simulink model "sampleModel646original"  (R2021b)
settings: Solver=VariableStepAuto  StartTime=0.0  StopTime=10.0  RelTol=1e-3
undefined symbols (not defined in the file): DiscIntNeverNeededParam, Newton, Raphson, sigbuilder_block
libraries: simulink x194, slpidlib x27
(part 4 of 5)

== system sampleModel646original/emi_2124 ==
  In1 : Inport
  emi_2125 : Inport  Port=2
  emi_2127 : slpidlib/PID Controller  Controller=PID  Form=Parallel  TimeDomain=Discrete-time  UseExternalTs=off  SampleTime=-1  IntegratorMethod=Forward Euler  FilterMethod=Forward Euler  ControllerParametersSource=internal  P=1  I=1  D=0  UseFilter=on  N=100  TunerSelectOption=Transfer Function Based (PID Tuner App)  InitialConditionSource=internal  InitialConditionForIntegrator=0  InitialConditionForFilter=0  DifferentiatorICPrevScaledInput=0  ExternalReset=none  TrackingMode=off  Kt=1  LimitOutput=off  SatLimitsSource=internal  UpperSaturationLimit=inf  LowerSaturationLimit=-inf  LinearizeAsGain=off  AntiWindupMode=none  Kb=1  POutMin=[]  POutMax=[]  IOutMin=[]  IOutMax=[]  DOutMin=[]  DOutMax=[]  NOutMin=[]  NOutMax=[]  SumOutMin=[]  SumOutMax=[]  SaturationOutMin=[]  SaturationOutMax=[]  PParamMin=[]  PParamMax=[]  IParamMin=[]  IParamMax=[]  DParamMin=[]  DParamMax=[]  NParamMin=[]  NParamMax=[]  KbParamMin=[]  KbParamMax=[]  KtParamMin=[]  KtParamMax=[]  KbOutMin=[]  KbOutMax=[]  KtOutMin=[]  KtOutMax=[]  IntegratorOutMin=[]  IntegratorOutMax=[]  FilterOutMin=[]  FilterOutMax=[]  SumI1OutMin=[]  SumI1OutMax=[]  SumI2OutMin=[]  SumI2OutMax=[]  SumI3OutMin=[]  SumI3OutMax=[]  SumI4OutMin=[]  SumI4OutMax=[]  SumDOutMin=[]  SumDOutMax=[]  DifferentiatorOutMin=[]  DifferentiatorOutMax=[]  FilterDiffOutCoefMin=[]  FilterDiffOutCoefMax=[]  ReciprocalOutMin=[]  ReciprocalOutMax=[]  SumDenOutMin=[]  SumDenOutMax=[]  SumNumOutMin=[]  SumNumOutMax=[]  DivideOutMin=[]  DivideOutMax=[]  UdiffTsProdOutMin=[]  UdiffTsProdOutMax=[]  NTsProdOutMin=[]  NTsProdOutMax=[]  UintegralTsProdOutMin=[]  UintegralTsProdOutMax=[]  UngainTsProdOutMin=[]  UngainTsProdOutMax=[]  IntegratorContinuousStateAttributes=''  IntegratorStateMustResolveToSignalObject=off  IntegratorRTWStateStorageClass=Auto  FilterContinuousStateAttributes=''  FilterStateMustResolveToSignalObject=off  FilterRTWStateStorageClass=Auto  ParallelPVariant=InternalParameters  IdealPVariant=Disabled  IVariant=InternalParameters  DVariant=InternalParameters  IntegratorVariant=Discrete  SatVariant=Disabled  AWVariant=Passthrough  PCopyVariant=Disabled  TRVariant=Disabled  FdbkBlocksVariant=Forward  IdealPFdbkVariant=Disabled  SatFdbkVariant=Disabled  DerivativeFilterVariant=ForwardEulerFilter  NVariant=InternalParameters  NCopyVariant=Disabled  FilterICVariant=InternalICsFilter  IntegratorICVariant=InternalICs  ExternalResetVariant=Disabled  TRSumVariant=Passthrough  SumFdbkVariant=Disabled  SumVariant=Sum_PID  TsampFilterVariant=InternalTs  TsampNgainVariant=Passthrough  TsampIntegralVariant=Passthrough  ExternalSaturationOutDataTypeStr=Inherit: Same as second input
  emi_2128 : simulink/Discrete/Difference  ICPrevInput=0.0  OutMin=[]  OutMax=[]  OutDataType=fixdt(1, 16)  OutScaling=2^-10  DoSatur=off
  emi_2129 : Sin  TimeSource=Use external signal  SampleTime=0
  emi_2130 : DiscreteZeroPole  Poles=[0 0.5]  Gain=1  SampleTime=-1
  emi_2131 : DiscreteZeroPole  Poles=[0 0.5]  Gain=1  SampleTime=-1
  emi_2132 : Math  SaturateOnIntegerOverflow=on
  emi_2133 : Rounding
  emi_2134 : simulink/Discontinuities/Rate Limiter Dynamic
  emi_2135 : simulink/Sources/Band-Limited White Noise  Cov=[0.1]  Ts=0.1  seed=[23341]
  Out1 : Outport
  emi_2126 : Outport  Port=2
  wires:
  In1/1 -> Out1/1
  emi_2127/1 -> emi_2128/1
  emi_2128/1 -> emi_2129/1
  emi_2129/1 -> emi_2130/1
  emi_2130/1 -> emi_2131/1
  emi_2131/1 -> emi_2132/1
  emi_2132/1 -> emi_2133/1
  emi_2133/1 -> emi_2134/1
  emi_2135/1 -> emi_2127/1
  emi_2134/1 -> emi_2126/1

== system sampleModel646original/emi_2143 ==
  emi_2150 : Inport
  Action Port : ActionPort  ActionPortLabel=if(0 > u1)
  emi_2147 : Math  SaturateOnIntegerOverflow=on
  emi_2148 : MinMax
  emi_2149 : Trigonometry
  emi_2152 : UnaryMinus
  emi_2153 : Gain
  emi_2154 : Trigonometry
  emi_2155 : Ground
  emi_2151 : Outport
  wires:
  emi_2150/1 -> emi_2147/1
  emi_2147/1 -> emi_2148/1
  emi_2148/1 -> emi_2149/1
  emi_2152/1 -> emi_2153/1
  emi_2153/1 -> emi_2154/1
  emi_2155/1 -> emi_2152/1
  emi_2154/1 -> emi_2151/1

== system sampleModel646original/emi_2158 ==
  In1 : Inport
  emi_2159 : Inport  Port=2
  emi_2161 : DiscreteStateSpace  SampleTime=-1
  emi_2162 : Relay
  emi_2163 : simulink/Discrete/Transfer Fcn First Order  PoleZ=0.95  ICPrevOutput=0.0  DoSatur=off
  emi_2164 : VariablePulseGenerator  SampleTime=0.1
  emi_2165 : Sum  Inputs=+
  emi_2166 : DiscreteTransferFcn
  emi_2167 : Sum  Inputs=+
  emi_2168 : Product  Inputs=*
  emi_2169 : simulink/Discontinuities/Wrap To Zero  Threshold=255
      settings: SourceProductBaseCode=SL
  emi_2170 : Quantizer
  emi_2171 : Sum  Inputs=+
  emi_2172 : DiscreteTransferFcn
  emi_2173 : simulink/Sources/Repeating Sequence Interpolated  OutValues=[3 1 4 2 1].'  TimeValues=[0 0.1 0.5 0.6 1].'  LookUpMeth=Interpolation-Use End Values  tsamp=0.01  OutMin=[]  OutMax=[]  OutDataTypeStr=double  OutputDataTypeScalingMode=double  OutDataType=fixdt(0,8)  OutScaling=2^-10
  Out1 : Outport
  emi_2160 : Outport  Port=2
  wires:
  In1/1 -> Out1/1
  emi_2161/1 -> emi_2162/1
  emi_2162/1 -> emi_2163/1
  emi_2163/1 -> emi_2164/1
  emi_2164/1 -> emi_2165/1
  emi_2165/1 -> emi_2166/1
  emi_2166/1 -> emi_2167/1
  emi_2167/1 -> emi_2168/1
  emi_2168/1 -> emi_2169/1
  emi_2169/1 -> emi_2170/1
  emi_2170/1 -> emi_2171/1
  emi_2171/1 -> emi_2172/1
  emi_2173/1 -> emi_2161/1
  emi_2172/1 -> emi_2160/1

== system sampleModel646original/emi_2180 ==
  emi_2187 : Inport
  Action Port : ActionPort  ActionPortLabel=if(0 > u1)
  emi_2184 : Trigonometry
  emi_2185 : Math  SaturateOnIntegerOverflow=on
  emi_2186 : MinMax
  emi_2189 : Sum  Inputs=+
  emi_2190 : Ground
  emi_2188 : Outport
  wires:
  emi_2187/1 -> emi_2184/1
  emi_2184/1 -> emi_2185/1
  emi_2185/1 -> emi_2186/1
  emi_2190/1 -> emi_2189/1
  emi_2189/1 -> emi_2188/1

== system sampleModel646original/emi_2193 ==
  In1 : Inport
  emi_2194 : Inport  Port=2
  emi_2196 : DiscreteStateSpace  SampleTime=-1
  emi_2197 : Product  Inputs=*
  emi_2198 : simulink/Discontinuities/Wrap To Zero  Threshold=255
      settings: SourceProductBaseCode=SL
  emi_2199 : simulink/Discrete/Transfer Fcn First Order  PoleZ=0.95  ICPrevOutput=0.0  DoSatur=off
  emi_2200 : simulink/Discontinuities/PWM  DisableCoverage=on  Period=1  DisallowZeroDutyCycle=off  RunAtFixedTimeIntervals=off  SampleTime=0.1
  emi_2201 : Rounding
  emi_2202 : DeadZone  SaturateOnIntegerOverflow=on
  emi_2203 : Clock
  Out1 : Outport
  emi_2195 : Outport  Port=2
  wires:
  In1/1 -> Out1/1
  emi_2196/1 -> emi_2197/1
  emi_2197/1 -> emi_2198/1
  emi_2198/1 -> emi_2199/1
  emi_2199/1 -> emi_2200/1
  emi_2200/1 -> emi_2201/1
  emi_2201/1 -> emi_2202/1
  emi_2203/1 -> emi_2196/1
  emi_2202/1 -> emi_2195/1

== system sampleModel646original/emi_22 ==
  In1 : Inport
  emi_23 : Inport  Port=2
  emi_25 : DiscreteZeroPole  Poles=[0 0.5]  Gain=1  SampleTime=-1
  emi_26 : simulink/Discontinuities/Saturation Dynamic  OutMin=[]  OutMax=[]  OutDataTypeStr=Inherit: Same as second input  OutDataType=fixdt(1, 16)  OutScaling=2^-10  DoSatur=off
  emi_27 : Sqrt  Operator=rSqrt  SaturateOnIntegerOverflow=on
  emi_28 : Relay
  emi_29 : simulink/Discontinuities/Wrap To Zero  Threshold=255
      settings: SourceProductBaseCode=SL
  emi_30 : VariablePulseGenerator  SampleTime=0.1
  emi_31 : Math  SaturateOnIntegerOverflow=on
  emi_32 : DiscreteZeroPole  Poles=[0 0.5]  Gain=1  SampleTime=-1
  emi_33 : DiscreteIntegrator  SampleTime=-1  ICPrevOutput=DiscIntNeverNeededParam  ICPrevScaledInput=DiscIntNeverNeededParam
  emi_34 : DiscreteTransferFcn
  emi_35 : VariablePulseGenerator  SampleTime=0.1
  emi_36 : simulink/Discrete/Transfer Fcn First Order  PoleZ=0.95  ICPrevOutput=0.0  DoSatur=off
  emi_37 : slpidlib/PID Controller  Controller=PID  Form=Parallel  TimeDomain=Discrete-time  UseExternalTs=off  SampleTime=-1  IntegratorMethod=Forward Euler  FilterMethod=Forward Euler  ControllerParametersSource=internal  P=1  I=1  D=0  UseFilter=on  N=100  TunerSelectOption=Transfer Function Based (PID Tuner App)  InitialConditionSource=internal  InitialConditionForIntegrator=0  InitialConditionForFilter=0  DifferentiatorICPrevScaledInput=0  ExternalReset=none  TrackingMode=off  Kt=1  LimitOutput=off  SatLimitsSource=internal  UpperSaturationLimit=inf  LowerSaturationLimit=-inf  LinearizeAsGain=off  AntiWindupMode=none  Kb=1  POutMin=[]  POutMax=[]  IOutMin=[]  IOutMax=[]  DOutMin=[]  DOutMax=[]  NOutMin=[]  NOutMax=[]  SumOutMin=[]  SumOutMax=[]  SaturationOutMin=[]  SaturationOutMax=[]  PParamMin=[]  PParamMax=[]  IParamMin=[]  IParamMax=[]  DParamMin=[]  DParamMax=[]  NParamMin=[]  NParamMax=[]  KbParamMin=[]  KbParamMax=[]  KtParamMin=[]  KtParamMax=[]  KbOutMin=[]  KbOutMax=[]  KtOutMin=[]  KtOutMax=[]  IntegratorOutMin=[]  IntegratorOutMax=[]  FilterOutMin=[]  FilterOutMax=[]  SumI1OutMin=[]  SumI1OutMax=[]  SumI2OutMin=[]  SumI2OutMax=[]  SumI3OutMin=[]  SumI3OutMax=[]  SumI4OutMin=[]  SumI4OutMax=[]  SumDOutMin=[]  SumDOutMax=[]  DifferentiatorOutMin=[]  DifferentiatorOutMax=[]  FilterDiffOutCoefMin=[]  FilterDiffOutCoefMax=[]  ReciprocalOutMin=[]  ReciprocalOutMax=[]  SumDenOutMin=[]  SumDenOutMax=[]  SumNumOutMin=[]  SumNumOutMax=[]  DivideOutMin=[]  DivideOutMax=[]  UdiffTsProdOutMin=[]  UdiffTsProdOutMax=[]  NTsProdOutMin=[]  NTsProdOutMax=[]  UintegralTsProdOutMin=[]  UintegralTsProdOutMax=[]  UngainTsProdOutMin=[]  UngainTsProdOutMax=[]  IntegratorContinuousStateAttributes=''  IntegratorStateMustResolveToSignalObject=off  IntegratorRTWStateStorageClass=Auto  FilterContinuousStateAttributes=''  FilterStateMustResolveToSignalObject=off  FilterRTWStateStorageClass=Auto  ParallelPVariant=InternalParameters  IdealPVariant=Disabled  IVariant=InternalParameters  DVariant=InternalParameters  IntegratorVariant=Discrete  SatVariant=Disabled  AWVariant=Passthrough  PCopyVariant=Disabled  TRVariant=Disabled  FdbkBlocksVariant=Forward  IdealPFdbkVariant=Disabled  SatFdbkVariant=Disabled  DerivativeFilterVariant=ForwardEulerFilter  NVariant=InternalParameters  NCopyVariant=Disabled  FilterICVariant=InternalICsFilter  IntegratorICVariant=InternalICs  ExternalResetVariant=Disabled  TRSumVariant=Passthrough  SumFdbkVariant=Disabled  SumVariant=Sum_PID  TsampFilterVariant=InternalTs  TsampNgainVariant=Passthrough  TsampIntegralVariant=Passthrough  ExternalSaturationOutDataTypeStr=Inherit: Same as second input
  emi_38 : Abs
  emi_39 : Sum  Inputs=+
  emi_40 : UnaryMinus
  emi_41 : Sin  TimeSource=Use external signal  SampleTime=0
  emi_42 : Math  SaturateOnIntegerOverflow=on
  emi_43 : slpidlib/PID Controller  Controller=PID  Form=Parallel  TimeDomain=Discrete-time  UseExternalTs=off  SampleTime=-1  IntegratorMethod=Forward Euler  FilterMethod=Forward Euler  ControllerParametersSource=internal  P=1  I=1  D=0  UseFilter=on  N=100  TunerSelectOption=Transfer Function Based (PID Tuner App)  InitialConditionSource=internal  InitialConditionForIntegrator=0  InitialConditionForFilter=0  DifferentiatorICPrevScaledInput=0  ExternalReset=none  TrackingMode=off  Kt=1  LimitOutput=off  SatLimitsSource=internal  UpperSaturationLimit=inf  LowerSaturationLimit=-inf  LinearizeAsGain=off  AntiWindupMode=none  Kb=1  POutMin=[]  POutMax=[]  IOutMin=[]  IOutMax=[]  DOutMin=[]  DOutMax=[]  NOutMin=[]  NOutMax=[]  SumOutMin=[]  SumOutMax=[]  SaturationOutMin=[]  SaturationOutMax=[]  PParamMin=[]  PParamMax=[]  IParamMin=[]  IParamMax=[]  DParamMin=[]  DParamMax=[]  NParamMin=[]  NParamMax=[]  KbParamMin=[]  KbParamMax=[]  KtParamMin=[]  KtParamMax=[]  KbOutMin=[]  KbOutMax=[]  KtOutMin=[]  KtOutMax=[]  IntegratorOutMin=[]  IntegratorOutMax=[]  FilterOutMin=[]  FilterOutMax=[]  SumI1OutMin=[]  SumI1OutMax=[]  SumI2OutMin=[]  SumI2OutMax=[]  SumI3OutMin=[]  SumI3OutMax=[]  SumI4OutMin=[]  SumI4OutMax=[]  SumDOutMin=[]  SumDOutMax=[]  DifferentiatorOutMin=[]  DifferentiatorOutMax=[]  FilterDiffOutCoefMin=[]  FilterDiffOutCoefMax=[]  ReciprocalOutMin=[]  ReciprocalOutMax=[]  SumDenOutMin=[]  SumDenOutMax=[]  SumNumOutMin=[]  SumNumOutMax=[]  DivideOutMin=[]  DivideOutMax=[]  UdiffTsProdOutMin=[]  UdiffTsProdOutMax=[]  NTsProdOutMin=[]  NTsProdOutMax=[]  UintegralTsProdOutMin=[]  UintegralTsProdOutMax=[]  UngainTsProdOutMin=[]  UngainTsProdOutMax=[]  IntegratorContinuousStateAttributes=''  IntegratorStateMustResolveToSignalObject=off  IntegratorRTWStateStorageClass=Auto  FilterContinuousStateAttributes=''  FilterStateMustResolveToSignalObject=off  FilterRTWStateStorageClass=Auto  ParallelPVariant=InternalParameters  IdealPVariant=Disabled  IVariant=InternalParameters  DVariant=InternalParameters  IntegratorVariant=Discrete  SatVariant=Disabled  AWVariant=Passthrough  PCopyVariant=Disabled  TRVariant=Disabled  FdbkBlocksVariant=Forward  IdealPFdbkVariant=Disabled  SatFdbkVariant=Disabled  DerivativeFilterVariant=ForwardEulerFilter  NVariant=InternalParameters  NCopyVariant=Disabled  FilterICVariant=InternalICsFilter  IntegratorICVariant=InternalICs  ExternalResetVariant=Disabled  TRSumVariant=Passthrough  SumFdbkVariant=Disabled  SumVariant=Sum_PID  TsampFilterVariant=InternalTs  TsampNgainVariant=Passthrough  TsampIntegralVariant=Passthrough  ExternalSaturationOutDataTypeStr=Inherit: Same as second input
  emi_44 : Math  SaturateOnIntegerOverflow=on
  emi_45 : slpidlib/PID Controller  Controller=PID  Form=Parallel  TimeDomain=Discrete-time  UseExternalTs=off  SampleTime=-1  IntegratorMethod=Forward Euler  FilterMethod=Forward Euler  ControllerParametersSource=internal  P=1  I=1  D=0  UseFilter=on  N=100  TunerSelectOption=Transfer Function Based (PID Tuner App)  InitialConditionSource=internal  InitialConditionForIntegrator=0  InitialConditionForFilter=0  DifferentiatorICPrevScaledInput=0  ExternalReset=none  TrackingMode=off  Kt=1  LimitOutput=off  SatLimitsSource=internal  UpperSaturationLimit=inf  LowerSaturationLimit=-inf  LinearizeAsGain=off  AntiWindupMode=none  Kb=1  POutMin=[]  POutMax=[]  IOutMin=[]  IOutMax=[]  DOutMin=[]  DOutMax=[]  NOutMin=[]  NOutMax=[]  SumOutMin=[]  SumOutMax=[]  SaturationOutMin=[]  SaturationOutMax=[]  PParamMin=[]  PParamMax=[]  IParamMin=[]  IParamMax=[]  DParamMin=[]  DParamMax=[]  NParamMin=[]  NParamMax=[]  KbParamMin=[]  KbParamMax=[]  KtParamMin=[]  KtParamMax=[]  KbOutMin=[]  KbOutMax=[]  KtOutMin=[]  KtOutMax=[]  IntegratorOutMin=[]  IntegratorOutMax=[]  FilterOutMin=[]  FilterOutMax=[]  SumI1OutMin=[]  SumI1OutMax=[]  SumI2OutMin=[]  SumI2OutMax=[]  SumI3OutMin=[]  SumI3OutMax=[]  SumI4OutMin=[]  SumI4OutMax=[]  SumDOutMin=[]  SumDOutMax=[]  DifferentiatorOutMin=[]  DifferentiatorOutMax=[]  FilterDiffOutCoefMin=[]  FilterDiffOutCoefMax=[]  ReciprocalOutMin=[]  ReciprocalOutMax=[]  SumDenOutMin=[]  SumDenOutMax=[]  SumNumOutMin=[]  SumNumOutMax=[]  DivideOutMin=[]  DivideOutMax=[]  UdiffTsProdOutMin=[]  UdiffTsProdOutMax=[]  NTsProdOutMin=[]  NTsProdOutMax=[]  UintegralTsProdOutMin=[]  UintegralTsProdOutMax=[]  UngainTsProdOutMin=[]  UngainTsProdOutMax=[]  IntegratorContinuousStateAttributes=''  IntegratorStateMustResolveToSignalObject=off  IntegratorRTWStateStorageClass=Auto  FilterContinuousStateAttributes=''  FilterStateMustResolveToSignalObject=off  FilterRTWStateStorageClass=Auto  ParallelPVariant=InternalParameters  IdealPVariant=Disabled  IVariant=InternalParameters  DVariant=InternalParameters  IntegratorVariant=Discrete  SatVariant=Disabled  AWVariant=Passthrough  PCopyVariant=Disabled  TRVariant=Disabled  FdbkBlocksVariant=Forward  IdealPFdbkVariant=Disabled  SatFdbkVariant=Disabled  DerivativeFilterVariant=ForwardEulerFilter  NVariant=InternalParameters  NCopyVariant=Disabled  FilterICVariant=InternalICsFilter  IntegratorICVariant=InternalICs  ExternalResetVariant=Disabled  TRSumVariant=Passthrough  SumFdbkVariant=Disabled  SumVariant=Sum_PID  TsampFilterVariant=InternalTs  TsampNgainVariant=Passthrough  TsampIntegralVariant=Passthrough  ExternalSaturationOutDataTypeStr=Inherit: Same as second input
  emi_46 : DiscreteFir
  emi_47 : VariablePulseGenerator  SampleTime=0.1
  emi_48 : Sum  Inputs=+
  emi_49 : simulink/Discrete/Transfer Fcn First Order  PoleZ=0.95  ICPrevOutput=0.0  DoSatur=off
  emi_50 : Quantizer
  emi_51 : DiscreteTransferFcn
  emi_52 : Sin  TimeSource=Use external signal  SampleTime=0
  emi_53 : simulink/Discontinuities/PWM  DisableCoverage=on  Period=1  DisallowZeroDutyCycle=off  RunAtFixedTimeIntervals=off  SampleTime=0.1
  emi_54 : simulink/Sources/Repeating Sequence  rep_seq_t=[0 2]  rep_seq_y=[0 2]
  Out1 : Outport
  emi_24 : Outport  Port=2
  wires:
  In1/1 -> Out1/1
  emi_25/1 -> emi_26/1
  emi_26/1 -> emi_27/1
  emi_27/1 -> emi_28/1
  emi_28/1 -> emi_29/1
  emi_29/1 -> emi_30/1
  emi_30/1 -> emi_31/1
  emi_31/1 -> emi_32/1
  emi_32/1 -> emi_33/1
  emi_33/1 -> emi_34/1
  emi_34/1 -> emi_35/1
  emi_35/1 -> emi_36/1
  emi_36/1 -> emi_37/1
  emi_37/1 -> emi_38/1
  emi_38/1 -> emi_39/1
  emi_39/1 -> emi_40/1
  emi_40/1 -> emi_41/1
  emi_41/1 -> emi_42/1
  emi_42/1 -> emi_43/1
  emi_43/1 -> emi_44/1
  emi_44/1 -> emi_45/1
  emi_45/1 -> emi_46/1
  emi_46/1 -> emi_47/1
  emi_47/1 -> emi_48/1
  emi_48/1 -> emi_49/1
  emi_49/1 -> emi_50/1
  emi_50/1 -> emi_51/1
  emi_51/1 -> emi_52/1
  emi_52/1 -> emi_53/1
  emi_54/1 -> emi_25/1
  emi_53/1 -> emi_24/1

== system sampleModel646original/emi_2210 ==
  emi_2217 : Inport
  Action Port : ActionPort  ActionPortLabel=if(0 > u1)
  emi_{2214,2216,2228,2238} (4 alike) : Gain
  emi_2215 : Abs
  emi_2219 : Trigonometry
  emi_2220 : Trigonometry
  emi_{2221,2223,2227,2233,2235,2239} (6 alike) : Sin  TimeSource=Use external signal  SampleTime=0
  emi_2222 : Product  Inputs=*
  emi_2224 : Math  SaturateOnIntegerOverflow=on
  emi_2225 : Math  SaturateOnIntegerOverflow=on
  emi_2226 : Sum  Inputs=+
  emi_2229 : MinMax
  emi_2230 : Product  Inputs=*
  emi_2231 : Sqrt  Operator=rSqrt  SaturateOnIntegerOverflow=on
  emi_2232 : Math  SaturateOnIntegerOverflow=on
  emi_2234 : Abs
  emi_2236 : Sum  Inputs=+
  emi_2237 : Sqrt  Operator=rSqrt  SaturateOnIntegerOverflow=on
  emi_2240 : Sum  Inputs=+
  emi_2241 : Ground
  emi_2218 : Outport
  wires:
  emi_2217/1 -> emi_2214/1
  emi_2214/1 -> emi_2215/1
  emi_2215/1 -> emi_2216/1
  emi_2219/1 -> emi_2220/1
  emi_2220/1 -> emi_2221/1
  emi_2221/1 -> emi_2222/1
  emi_2222/1 -> emi_2223/1
  emi_2223/1 -> emi_2224/1
  emi_2224/1 -> emi_2225/1
  emi_2225/1 -> emi_2226/1
  emi_2226/1 -> emi_2227/1
  emi_2227/1 -> emi_2228/1
  emi_2228/1 -> emi_2229/1
  emi_2229/1 -> emi_2230/1
  emi_2230/1 -> emi_2231/1
  emi_2231/1 -> emi_2232/1
  emi_2232/1 -> emi_2233/1
  emi_2233/1 -> emi_2234/1
  emi_2234/1 -> emi_2235/1
  emi_2235/1 -> emi_2236/1
  emi_2236/1 -> emi_2237/1
  emi_2237/1 -> emi_2238/1
  emi_2238/1 -> emi_2239/1
  emi_2239/1 -> emi_2240/1
  emi_2241/1 -> emi_2219/1
  emi_2240/1 -> emi_2218/1

== system sampleModel646original/emi_2244 ==
  In1 : Inport
  emi_2245 : Inport  Port=2
  emi_2247 : UnaryMinus
  emi_2248 : simulink/Discontinuities/Saturation Dynamic  OutMin=[]  OutMax=[]  OutDataTypeStr=Inherit: Same as second input  OutDataType=fixdt(1, 16)  OutScaling=2^-10  DoSatur=off
  emi_2249 : Product  Inputs=*
  emi_2250 : Abs
  emi_2251 : simulink/Discontinuities/Saturation Dynamic  OutMin=[]  OutMax=[]  OutDataTypeStr=Inherit: Same as second input  OutDataType=fixdt(1, 16)  OutScaling=2^-10  DoSatur=off
  emi_2252 : slpidlib/PID Controller  Controller=PID  Form=Parallel  TimeDomain=Discrete-time  UseExternalTs=off  SampleTime=-1  IntegratorMethod=Forward Euler  FilterMethod=Forward Euler  ControllerParametersSource=internal  P=1  I=1  D=0  UseFilter=on  N=100  TunerSelectOption=Transfer Function Based (PID Tuner App)  InitialConditionSource=internal  InitialConditionForIntegrator=0  InitialConditionForFilter=0  DifferentiatorICPrevScaledInput=0  ExternalReset=none  TrackingMode=off  Kt=1  LimitOutput=off  SatLimitsSource=internal  UpperSaturationLimit=inf  LowerSaturationLimit=-inf  LinearizeAsGain=off  AntiWindupMode=none  Kb=1  POutMin=[]  POutMax=[]  IOutMin=[]  IOutMax=[]  DOutMin=[]  DOutMax=[]  NOutMin=[]  NOutMax=[]  SumOutMin=[]  SumOutMax=[]  SaturationOutMin=[]  SaturationOutMax=[]  PParamMin=[]  PParamMax=[]  IParamMin=[]  IParamMax=[]  DParamMin=[]  DParamMax=[]  NParamMin=[]  NParamMax=[]  KbParamMin=[]  KbParamMax=[]  KtParamMin=[]  KtParamMax=[]  KbOutMin=[]  KbOutMax=[]  KtOutMin=[]  KtOutMax=[]  IntegratorOutMin=[]  IntegratorOutMax=[]  FilterOutMin=[]  FilterOutMax=[]  SumI1OutMin=[]  SumI1OutMax=[]  SumI2OutMin=[]  SumI2OutMax=[]  SumI3OutMin=[]  SumI3OutMax=[]  SumI4OutMin=[]  SumI4OutMax=[]  SumDOutMin=[]  SumDOutMax=[]  DifferentiatorOutMin=[]  DifferentiatorOutMax=[]  FilterDiffOutCoefMin=[]  FilterDiffOutCoefMax=[]  ReciprocalOutMin=[]  ReciprocalOutMax=[]  SumDenOutMin=[]  SumDenOutMax=[]  SumNumOutMin=[]  SumNumOutMax=[]  DivideOutMin=[]  DivideOutMax=[]  UdiffTsProdOutMin=[]  UdiffTsProdOutMax=[]  NTsProdOutMin=[]  NTsProdOutMax=[]  UintegralTsProdOutMin=[]  UintegralTsProdOutMax=[]  UngainTsProdOutMin=[]  UngainTsProdOutMax=[]  IntegratorContinuousStateAttributes=''  IntegratorStateMustResolveToSignalObject=off  IntegratorRTWStateStorageClass=Auto  FilterContinuousStateAttributes=''  FilterStateMustResolveToSignalObject=off  FilterRTWStateStorageClass=Auto  ParallelPVariant=InternalParameters  IdealPVariant=Disabled  IVariant=InternalParameters  DVariant=InternalParameters  IntegratorVariant=Discrete  SatVariant=Disabled  AWVariant=Passthrough  PCopyVariant=Disabled  TRVariant=Disabled  FdbkBlocksVariant=Forward  IdealPFdbkVariant=Disabled  SatFdbkVariant=Disabled  DerivativeFilterVariant=ForwardEulerFilter  NVariant=InternalParameters  NCopyVariant=Disabled  FilterICVariant=InternalICsFilter  IntegratorICVariant=InternalICs  ExternalResetVariant=Disabled  TRSumVariant=Passthrough  SumFdbkVariant=Disabled  SumVariant=Sum_PID  TsampFilterVariant=InternalTs  TsampNgainVariant=Passthrough  TsampIntegralVariant=Passthrough  ExternalSaturationOutDataTypeStr=Inherit: Same as second input
  emi_2253 : Trigonometry
  emi_2254 : DiscreteFir
  emi_2255 : Rounding
  emi_2256 : Rounding
  emi_2257 : Rounding
  emi_2258 : DiscreteTransferFcn
  emi_2259 : Relay
  emi_2260 : Sin  TimeSource=Use external signal  SampleTime=0
  emi_2261 : simulink/Sources/Repeating Sequence Stair  OutValues=[3 1 4 2 1].'  tsamp=-1  OutMin=[]  OutMax=[]  OutDataTypeStr=double  OutputDataTypeScalingMode=double  OutDataType=fixdt(0,8)  ConRadixGroup=Best Precision: Vector-wise  OutScaling=2^-12
  Out1 : Outport
  emi_2246 : Outport  Port=2
  wires:
  In1/1 -> Out1/1
  emi_2247/1 -> emi_2248/1
  emi_2248/1 -> emi_2249/1
  emi_2249/1 -> emi_2250/1
  emi_2250/1 -> emi_2251/1
  emi_2251/1 -> emi_2252/1
  emi_2252/1 -> emi_2253/1
  emi_2253/1 -> emi_2254/1
  emi_2254/1 -> emi_2255/1
  emi_2255/1 -> emi_2256/1
  emi_2256/1 -> emi_2257/1
  emi_2257/1 -> emi_2258/1
  emi_2258/1 -> emi_2259/1
  emi_2259/1 -> emi_2260/1
  emi_2261/1 -> emi_2247/1
  emi_2260/1 -> emi_2246/1

== system sampleModel646original/emi_231 ==
  In1 : Inport
  emi_232 : Inport  Port=2
  emi_234 : Relay
  emi_235 : simulink/Discontinuities/Rate Limiter Dynamic
  emi_236 : DiscreteZeroPole  Poles=[0 0.5]  Gain=1  SampleTime=-1
  emi_237 : slpidlib/PID Controller  Controller=PID  Form=Parallel  TimeDomain=Discrete-time  UseExternalTs=off  SampleTime=-1  IntegratorMethod=Forward Euler  FilterMethod=Forward Euler  ControllerParametersSource=internal  P=1  I=1  D=0  UseFilter=on  N=100  TunerSelectOption=Transfer Function Based (PID Tuner App)  InitialConditionSource=internal  InitialConditionForIntegrator=0  InitialConditionForFilter=0  DifferentiatorICPrevScaledInput=0  ExternalReset=none  TrackingMode=off  Kt=1  LimitOutput=off  SatLimitsSource=internal  UpperSaturationLimit=inf  LowerSaturationLimit=-inf  LinearizeAsGain=off  AntiWindupMode=none  Kb=1  POutMin=[]  POutMax=[]  IOutMin=[]  IOutMax=[]  DOutMin=[]  DOutMax=[]  NOutMin=[]  NOutMax=[]  SumOutMin=[]  SumOutMax=[]  SaturationOutMin=[]  SaturationOutMax=[]  PParamMin=[]  PParamMax=[]  IParamMin=[]  IParamMax=[]  DParamMin=[]  DParamMax=[]  NParamMin=[]  NParamMax=[]  KbParamMin=[]  KbParamMax=[]  KtParamMin=[]  KtParamMax=[]  KbOutMin=[]  KbOutMax=[]  KtOutMin=[]  KtOutMax=[]  IntegratorOutMin=[]  IntegratorOutMax=[]  FilterOutMin=[]  FilterOutMax=[]  SumI1OutMin=[]  SumI1OutMax=[]  SumI2OutMin=[]  SumI2OutMax=[]  SumI3OutMin=[]  SumI3OutMax=[]  SumI4OutMin=[]  SumI4OutMax=[]  SumDOutMin=[]  SumDOutMax=[]  DifferentiatorOutMin=[]  DifferentiatorOutMax=[]  FilterDiffOutCoefMin=[]  FilterDiffOutCoefMax=[]  ReciprocalOutMin=[]  ReciprocalOutMax=[]  SumDenOutMin=[]  SumDenOutMax=[]  SumNumOutMin=[]  SumNumOutMax=[]  DivideOutMin=[]  DivideOutMax=[]  UdiffTsProdOutMin=[]  UdiffTsProdOutMax=[]  NTsProdOutMin=[]  NTsProdOutMax=[]  UintegralTsProdOutMin=[]  UintegralTsProdOutMax=[]  UngainTsProdOutMin=[]  UngainTsProdOutMax=[]  IntegratorContinuousStateAttributes=''  IntegratorStateMustResolveToSignalObject=off  IntegratorRTWStateStorageClass=Auto  FilterContinuousStateAttributes=''  FilterStateMustResolveToSignalObject=off  FilterRTWStateStorageClass=Auto  ParallelPVariant=InternalParameters  IdealPVariant=Disabled  IVariant=InternalParameters  DVariant=InternalParameters  IntegratorVariant=Discrete  SatVariant=Disabled  AWVariant=Passthrough  PCopyVariant=Disabled  TRVariant=Disabled  FdbkBlocksVariant=Forward  IdealPFdbkVariant=Disabled  SatFdbkVariant=Disabled  DerivativeFilterVariant=ForwardEulerFilter  NVariant=InternalParameters  NCopyVariant=Disabled  FilterICVariant=InternalICsFilter  IntegratorICVariant=InternalICs  ExternalResetVariant=Disabled  TRSumVariant=Passthrough  SumFdbkVariant=Disabled  SumVariant=Sum_PID  TsampFilterVariant=InternalTs  TsampNgainVariant=Passthrough  TsampIntegralVariant=Passthrough  ExternalSaturationOutDataTypeStr=Inherit: Same as second input
  emi_238 : VariablePulseGenerator  SampleTime=0.1
  emi_239 : DiscreteStateSpace  SampleTime=-1
  emi_240 : Product  Inputs=*
  emi_241 : Sin  TimeSource=Use external signal  SampleTime=0
  emi_242 : Rounding
  emi_243 : MinMax
  emi_244 : simulink/Discrete/Transfer Fcn First Order  PoleZ=0.95  ICPrevOutput=0.0  DoSatur=off
  emi_245 : simulink/Discontinuities/Wrap To Zero  Threshold=255
      settings: SourceProductBaseCode=SL
  emi_246 : Math  SaturateOnIntegerOverflow=on
  emi_247 : simulink/Sources/Repeating Sequence Stair  OutValues=[3 1 4 2 1].'  tsamp=-1  OutMin=[]  OutMax=[]  OutDataTypeStr=double  OutputDataTypeScalingMode=double  OutDataType=fixdt(0,8)  ConRadixGroup=Best Precision: Vector-wise  OutScaling=2^-12
  Out1 : Outport
  emi_233 : Outport  Port=2
  wires:
  In1/1 -> Out1/1
  emi_234/1 -> emi_235/1
  emi_235/1 -> emi_236/1
  emi_236/1 -> emi_237/1
  emi_237/1 -> emi_238/1
  emi_238/1 -> emi_239/1
  emi_239/1 -> emi_240/1
  emi_240/1 -> emi_241/1
  emi_241/1 -> emi_242/1
  emi_242/1 -> emi_243/1
  emi_243/1 -> emi_244/1
  emi_244/1 -> emi_245/1
  emi_245/1 -> emi_246/1
  emi_247/1 -> emi_234/1
  emi_246/1 -> emi_233/1

== system sampleModel646original/emi_254 ==
  emi_261 : Inport
  Action Port : ActionPort  ActionPortLabel=if(-1.617560e+02 > u1)
  emi_258 : Trigonometry  SampleTime=1
  emi_259 : Math  SampleTime=1  SaturateOnIntegerOverflow=on
  emi_260 : Abs  SampleTime=1
  emi_263 : Abs
  emi_{264,270..271,275,287..288} (6 alike) : Product  Inputs=*
  emi_{265,284,286,289} (4 alike) : Sin  TimeSource=Use external signal  SampleTime=0
  emi_266 : UnaryMinus
  emi_267 : Abs
  emi_268 : UnaryMinus
  emi_{269,279..280,283,285,290} (6 alike) : Sqrt  Operator=rSqrt  SaturateOnIntegerOverflow=on
  emi_272 : MinMax
  emi_273 : Sum  Inputs=+
  emi_274 : UnaryMinus
  emi_276 : Sum  Inputs=+
  emi_277 : Math  SaturateOnIntegerOverflow=on
  emi_278 : Math  SaturateOnIntegerOverflow=on
  emi_281 : Abs
  emi_282 : Rounding
  emi_291 : MinMax
  emi_292 : MinMax
  emi_293 : Gain
  emi_294 : Gain
  emi_295 : Ground
  emi_262 : Outport
  wires:
  emi_261/1 -> emi_258/1
  emi_258/1 -> emi_259/1
  emi_259/1 -> emi_260/1
  emi_263/1 -> emi_264/1
  emi_264/1 -> emi_265/1
  emi_265/1 -> emi_266/1
  emi_266/1 -> emi_267/1
  emi_267/1 -> emi_268/1
  emi_268/1 -> emi_269/1
  emi_269/1 -> emi_270/1
  emi_270/1 -> emi_271/1
  emi_271/1 -> emi_272/1
  emi_272/1 -> emi_273/1
  emi_273/1 -> emi_274/1
  emi_274/1 -> emi_275/1
  emi_275/1 -> emi_276/1
  emi_276/1 -> emi_277/1
  emi_277/1 -> emi_278/1
  emi_278/1 -> emi_279/1
  emi_279/1 -> emi_280/1
  emi_280/1 -> emi_281/1
  emi_281/1 -> emi_282/1
  emi_282/1 -> emi_283/1
  emi_283/1 -> emi_284/1
  emi_284/1 -> emi_285/1
  emi_285/1 -> emi_286/1
  emi_286/1 -> emi_287/1
  emi_287/1 -> emi_288/1
  emi_288/1 -> emi_289/1
  emi_289/1 -> emi_290/1
  emi_290/1 -> emi_291/1
  emi_291/1 -> emi_292/1
  emi_292/1 -> emi_293/1
  emi_293/1 -> emi_294/1
  emi_295/1 -> emi_263/1
  emi_294/1 -> emi_262/1

== system sampleModel646original/emi_298 ==
  In1 : Inport
  emi_299 : Inport  Port=2
  emi_301 : DiscreteStateSpace  SampleTime=-1
  emi_302 : Math  SaturateOnIntegerOverflow=on
  emi_303 : Trigonometry
  emi_304 : simulink/Discontinuities/Rate Limiter Dynamic
  emi_305 : Quantizer
  emi_306 : VariablePulseGenerator  SampleTime=0.1
  emi_307 : DiscreteFir
  emi_308 : DiscreteTransferFcn
  emi_309 : Rounding
  emi_310 : DiscreteZeroPole  Poles=[0 0.5]  Gain=1  SampleTime=-1
  emi_311 : DiscreteFilter
  emi_312 : DeadZone  SaturateOnIntegerOverflow=on
  emi_313 : simulink/Discrete/Difference  ICPrevInput=0.0  OutMin=[]  OutMax=[]  OutDataType=fixdt(1, 16)  OutScaling=2^-10  DoSatur=off
  emi_314 : Sin  TimeSource=Use external signal  SampleTime=0
  emi_315 : DeadZone  SaturateOnIntegerOverflow=on
  emi_316 : Rounding
  emi_317 : Product  Inputs=*
  emi_318 : slpidlib/PID Controller  Controller=PID  Form=Parallel  TimeDomain=Discrete-time  UseExternalTs=off  SampleTime=-1  IntegratorMethod=Forward Euler  FilterMethod=Forward Euler  ControllerParametersSource=internal  P=1  I=1  D=0  UseFilter=on  N=100  TunerSelectOption=Transfer Function Based (PID Tuner App)  InitialConditionSource=internal  InitialConditionForIntegrator=0  InitialConditionForFilter=0  DifferentiatorICPrevScaledInput=0  ExternalReset=none  TrackingMode=off  Kt=1  LimitOutput=off  SatLimitsSource=internal  UpperSaturationLimit=inf  LowerSaturationLimit=-inf  LinearizeAsGain=off  AntiWindupMode=none  Kb=1  POutMin=[]  POutMax=[]  IOutMin=[]  IOutMax=[]  DOutMin=[]  DOutMax=[]  NOutMin=[]  NOutMax=[]  SumOutMin=[]  SumOutMax=[]  SaturationOutMin=[]  SaturationOutMax=[]  PParamMin=[]  PParamMax=[]  IParamMin=[]  IParamMax=[]  DParamMin=[]  DParamMax=[]  NParamMin=[]  NParamMax=[]  KbParamMin=[]  KbParamMax=[]  KtParamMin=[]  KtParamMax=[]  KbOutMin=[]  KbOutMax=[]  KtOutMin=[]  KtOutMax=[]  IntegratorOutMin=[]  IntegratorOutMax=[]  FilterOutMin=[]  FilterOutMax=[]  SumI1OutMin=[]  SumI1OutMax=[]  SumI2OutMin=[]  SumI2OutMax=[]  SumI3OutMin=[]  SumI3OutMax=[]  SumI4OutMin=[]  SumI4OutMax=[]  SumDOutMin=[]  SumDOutMax=[]  DifferentiatorOutMin=[]  DifferentiatorOutMax=[]  FilterDiffOutCoefMin=[]  FilterDiffOutCoefMax=[]  ReciprocalOutMin=[]  ReciprocalOutMax=[]  SumDenOutMin=[]  SumDenOutMax=[]  SumNumOutMin=[]  SumNumOutMax=[]  DivideOutMin=[]  DivideOutMax=[]  UdiffTsProdOutMin=[]  UdiffTsProdOutMax=[]  NTsProdOutMin=[]  NTsProdOutMax=[]  UintegralTsProdOutMin=[]  UintegralTsProdOutMax=[]  UngainTsProdOutMin=[]  UngainTsProdOutMax=[]  IntegratorContinuousStateAttributes=''  IntegratorStateMustResolveToSignalObject=off  IntegratorRTWStateStorageClass=Auto  FilterContinuousStateAttributes=''  FilterStateMustResolveToSignalObject=off  FilterRTWStateStorageClass=Auto  ParallelPVariant=InternalParameters  IdealPVariant=Disabled  IVariant=InternalParameters  DVariant=InternalParameters  IntegratorVariant=Discrete  SatVariant=Disabled  AWVariant=Passthrough  PCopyVariant=Disabled  TRVariant=Disabled  FdbkBlocksVariant=Forward  IdealPFdbkVariant=Disabled  SatFdbkVariant=Disabled  DerivativeFilterVariant=ForwardEulerFilter  NVariant=InternalParameters  NCopyVariant=Disabled  FilterICVariant=InternalICsFilter  IntegratorICVariant=InternalICs  ExternalResetVariant=Disabled  TRSumVariant=Passthrough  SumFdbkVariant=Disabled  SumVariant=Sum_PID  TsampFilterVariant=InternalTs  TsampNgainVariant=Passthrough  TsampIntegralVariant=Passthrough  ExternalSaturationOutDataTypeStr=Inherit: Same as second input
  emi_319 : Sum  Inputs=+
  emi_320 : Rounding
  emi_321 : slpidlib/PID Controller  Controller=PID  Form=Parallel  TimeDomain=Discrete-time  UseExternalTs=off  SampleTime=-1  IntegratorMethod=Forward Euler  FilterMethod=Forward Euler  ControllerParametersSource=internal  P=1  I=1  D=0  UseFilter=on  N=100  TunerSelectOption=Transfer Function Based (PID Tuner App)  InitialConditionSource=internal  InitialConditionForIntegrator=0  InitialConditionForFilter=0  DifferentiatorICPrevScaledInput=0  ExternalReset=none  TrackingMode=off  Kt=1  LimitOutput=off  SatLimitsSource=internal  UpperSaturationLimit=inf  LowerSaturationLimit=-inf  LinearizeAsGain=off  AntiWindupMode=none  Kb=1  POutMin=[]  POutMax=[]  IOutMin=[]  IOutMax=[]  DOutMin=[]  DOutMax=[]  NOutMin=[]  NOutMax=[]  SumOutMin=[]  SumOutMax=[]  SaturationOutMin=[]  SaturationOutMax=[]  PParamMin=[]  PParamMax=[]  IParamMin=[]  IParamMax=[]  DParamMin=[]  DParamMax=[]  NParamMin=[]  NParamMax=[]  KbParamMin=[]  KbParamMax=[]  KtParamMin=[]  KtParamMax=[]  KbOutMin=[]  KbOutMax=[]  KtOutMin=[]  KtOutMax=[]  IntegratorOutMin=[]  IntegratorOutMax=[]  FilterOutMin=[]  FilterOutMax=[]  SumI1OutMin=[]  SumI1OutMax=[]  SumI2OutMin=[]  SumI2OutMax=[]  SumI3OutMin=[]  SumI3OutMax=[]  SumI4OutMin=[]  SumI4OutMax=[]  SumDOutMin=[]  SumDOutMax=[]  DifferentiatorOutMin=[]  DifferentiatorOutMax=[]  FilterDiffOutCoefMin=[]  FilterDiffOutCoefMax=[]  ReciprocalOutMin=[]  ReciprocalOutMax=[]  SumDenOutMin=[]  SumDenOutMax=[]  SumNumOutMin=[]  SumNumOutMax=[]  DivideOutMin=[]  DivideOutMax=[]  UdiffTsProdOutMin=[]  UdiffTsProdOutMax=[]  NTsProdOutMin=[]  NTsProdOutMax=[]  UintegralTsProdOutMin=[]  UintegralTsProdOutMax=[]  UngainTsProdOutMin=[]  UngainTsProdOutMax=[]  IntegratorContinuousStateAttributes=''  IntegratorStateMustResolveToSignalObject=off  IntegratorRTWStateStorageClass=Auto  FilterContinuousStateAttributes=''  FilterStateMustResolveToSignalObject=off  FilterRTWStateStorageClass=Auto  ParallelPVariant=InternalParameters  IdealPVariant=Disabled  IVariant=InternalParameters  DVariant=InternalParameters  IntegratorVariant=Discrete  SatVariant=Disabled  AWVariant=Passthrough  PCopyVariant=Disabled  TRVariant=Disabled  FdbkBlocksVariant=Forward  IdealPFdbkVariant=Disabled  SatFdbkVariant=Disabled  DerivativeFilterVariant=ForwardEulerFilter  NVariant=InternalParameters  NCopyVariant=Disabled  FilterICVariant=InternalICsFilter  IntegratorICVariant=InternalICs  ExternalResetVariant=Disabled  TRSumVariant=Passthrough  SumFdbkVariant=Disabled  SumVariant=Sum_PID  TsampFilterVariant=InternalTs  TsampNgainVariant=Passthrough  TsampIntegralVariant=Passthrough  ExternalSaturationOutDataTypeStr=Inherit: Same as second input
  emi_322 : Gain
  emi_323 : simulink/Discrete/Discrete Derivative  gainval=1.0  ICPrevScaledInput=0.0  OutMin=[]  OutMax=[]  OutDataType=fixdt(1, 16)  OutScaling=2^-10  DoSatur=off
  emi_324 : simulink/Discrete/Transfer Fcn First Order  PoleZ=0.95  ICPrevOutput=0.0  DoSatur=off
  emi_325 : Ground
  Out1 : Outport
  emi_300 : Outport  Port=2
  wires:
  In1/1 -> Out1/1
  emi_301/1 -> emi_302/1
  emi_302/1 -> emi_303/1
  emi_303/1 -> emi_304/1
  emi_304/1 -> emi_305/1
  emi_305/1 -> emi_306/1
  emi_306/1 -> emi_307/1
  emi_307/1 -> emi_308/1
  emi_308/1 -> emi_309/1
  emi_309/1 -> emi_310/1
  emi_310/1 -> emi_311/1
  emi_311/1 -> emi_312/1
  emi_312/1 -> emi_313/1
  emi_313/1 -> emi_314/1
  emi_314/1 -> emi_315/1
  emi_315/1 -> emi_316/1
  emi_316/1 -> emi_317/1
  emi_317/1 -> emi_318/1
  emi_318/1 -> emi_319/1
  emi_319/1 -> emi_320/1
  emi_320/1 -> emi_321/1
  emi_321/1 -> emi_322/1
  emi_322/1 -> emi_323/1
  emi_323/1 -> emi_324/1
  emi_325/1 -> emi_301/1
  emi_324/1 -> emi_300/1

== system sampleModel646original/emi_3 ==
  emi_10 : Inport
  Action Port : ActionPort  ActionPortLabel=if(-1.382844e+09 > u1)
  emi_12 : Sin  TimeSource=Use external signal  SampleTime=0
  emi_13 : Sum  Inputs=+
  emi_14 : Sqrt  Operator=rSqrt  SaturateOnIntegerOverflow=on
  emi_15 : Sin  TimeSource=Use external signal  SampleTime=0
  emi_16 : Trigonometry
  emi_17 : Sin  TimeSource=Use external signal  SampleTime=0
  emi_18 : Gain
  emi_19 : Ground
  emi_7 : Math  SampleTime=1  SaturateOnIntegerOverflow=on
  emi_8 : Abs  SampleTime=1
  emi_9 : Gain  SampleTime=1
  emi_11 : Outport
  wires:
  emi_10/1 -> emi_7/1
  emi_7/1 -> emi_8/1
  emi_8/1 -> emi_9/1
  emi_12/1 -> emi_13/1
  emi_13/1 -> emi_14/1
  emi_14/1 -> emi_15/1
  emi_15/1 -> emi_16/1
  emi_16/1 -> emi_17/1
  emi_17/1 -> emi_18/1
  emi_19/1 -> emi_12/1
  emi_18/1 -> emi_11/1

== system sampleModel646original/emi_332 ==
  emi_339 : Inport
  Action Port : ActionPort  ActionPortLabel=if(0 > u1)
  emi_336 : Gain  SampleTime=0
  emi_337 : MinMax  SampleTime=0
  emi_338 : Gain  SampleTime=0
  emi_341 : Sum  Inputs=+
  emi_{342,346,350,359} (4 alike) : Math  SaturateOnIntegerOverflow=on
  emi_343 : Trigonometry
  emi_344 : Trigonometry
  emi_345 : Trigonometry
  emi_347 : Product  Inputs=*
  emi_348 : Sin  TimeSource=Use external signal  SampleTime=0
  emi_349 : MinMax
  emi_351 : Gain
  emi_352 : Sqrt  Operator=rSqrt  SaturateOnIntegerOverflow=on
  emi_{353,357..358,363} (4 alike) : UnaryMinus
  emi_354 : MinMax
  emi_355 : Sqrt  Operator=rSqrt  SaturateOnIntegerOverflow=on
  emi_356 : Sin  TimeSource=Use external signal  SampleTime=0
  emi_360 : Product  Inputs=*
  emi_361 : Sin  TimeSource=Use external signal  SampleTime=0
  emi_362 : Abs
  emi_364 : Ground
  emi_340 : Outport
  wires:
  emi_339/1 -> emi_336/1
  emi_336/1 -> emi_337/1
  emi_337/1 -> emi_338/1
  emi_341/1 -> emi_342/1
  emi_342/1 -> emi_343/1
  emi_343/1 -> emi_344/1
  emi_344/1 -> emi_345/1
  emi_345/1 -> emi_346/1
  emi_346/1 -> emi_347/1
  emi_347/1 -> emi_348/1
  emi_348/1 -> emi_349/1
  emi_349/1 -> emi_350/1
  emi_350/1 -> emi_351/1
  emi_351/1 -> emi_352/1
  emi_352/1 -> emi_353/1
  emi_353/1 -> emi_354/1
  emi_354/1 -> emi_355/1
  emi_355/1 -> emi_356/1
  emi_356/1 -> emi_357/1
  emi_357/1 -> emi_358/1
  emi_358/1 -> emi_359/1
  emi_359/1 -> emi_360/1
  emi_360/1 -> emi_361/1
  emi_361/1 -> emi_362/1
  emi_362/1 -> emi_363/1
  emi_364/1 -> emi_341/1
  emi_363/1 -> emi_340/1

== system sampleModel646original/emi_367 ==
  In1 : Inport
  emi_368 : Inport  Port=2
  emi_{370,379,388,392} (4 alike) : simulink/Discrete/Transfer Fcn First Order  PoleZ=0.95  ICPrevOutput=0.0  DoSatur=off
  emi_371 : Sin  TimeSource=Use external signal  SampleTime=0
  emi_372 : simulink/Discontinuities/Rate Limiter Dynamic
  emi_373 : DiscreteTransferFcn
  emi_374 : Math  SaturateOnIntegerOverflow=on
  emi_375 : simulink/Discrete/Difference  ICPrevInput=0.0  OutMin=[]  OutMax=[]  OutDataType=fixdt(1, 16)  OutScaling=2^-10  DoSatur=off
  emi_376 : Quantizer
  emi_377 : DiscreteZeroPole  Poles=[0 0.5]  Gain=1  SampleTime=-1
  emi_378 : Gain
  emi_380 : DeadZone  SaturateOnIntegerOverflow=on
  emi_381 : DiscreteTransferFcn
  emi_382 : Product  Inputs=*
  emi_383 : Math  SaturateOnIntegerOverflow=on
  emi_384 : VariablePulseGenerator  SampleTime=0.1
  emi_385 : simulink/Discrete/Difference  ICPrevInput=0.0  OutMin=[]  OutMax=[]  OutDataType=fixdt(1, 16)  OutScaling=2^-10  DoSatur=off
  emi_386 : Sum  Inputs=+
  emi_387 : slpidlib/PID Controller  Controller=PID  Form=Parallel  TimeDomain=Discrete-time  UseExternalTs=off  SampleTime=-1  IntegratorMethod=Forward Euler  FilterMethod=Forward Euler  ControllerParametersSource=internal  P=1  I=1  D=0  UseFilter=on  N=100  TunerSelectOption=Transfer Function Based (PID Tuner App)  InitialConditionSource=internal  InitialConditionForIntegrator=0  InitialConditionForFilter=0  DifferentiatorICPrevScaledInput=0  ExternalReset=none  TrackingMode=off  Kt=1  LimitOutput=off  SatLimitsSource=internal  UpperSaturationLimit=inf  LowerSaturationLimit=-inf  LinearizeAsGain=off  AntiWindupMode=none  Kb=1  POutMin=[]  POutMax=[]  IOutMin=[]  IOutMax=[]  DOutMin=[]  DOutMax=[]  NOutMin=[]  NOutMax=[]  SumOutMin=[]  SumOutMax=[]  SaturationOutMin=[]  SaturationOutMax=[]  PParamMin=[]  PParamMax=[]  IParamMin=[]  IParamMax=[]  DParamMin=[]  DParamMax=[]  NParamMin=[]  NParamMax=[]  KbParamMin=[]  KbParamMax=[]  KtParamMin=[]  KtParamMax=[]  KbOutMin=[]  KbOutMax=[]  KtOutMin=[]  KtOutMax=[]  IntegratorOutMin=[]  IntegratorOutMax=[]  FilterOutMin=[]  FilterOutMax=[]  SumI1OutMin=[]  SumI1OutMax=[]  SumI2OutMin=[]  SumI2OutMax=[]  SumI3OutMin=[]  SumI3OutMax=[]  SumI4OutMin=[]  SumI4OutMax=[]  SumDOutMin=[]  SumDOutMax=[]  DifferentiatorOutMin=[]  DifferentiatorOutMax=[]  FilterDiffOutCoefMin=[]  FilterDiffOutCoefMax=[]  ReciprocalOutMin=[]  ReciprocalOutMax=[]  SumDenOutMin=[]  SumDenOutMax=[]  SumNumOutMin=[]  SumNumOutMax=[]  DivideOutMin=[]  DivideOutMax=[]  UdiffTsProdOutMin=[]  UdiffTsProdOutMax=[]  NTsProdOutMin=[]  NTsProdOutMax=[]  UintegralTsProdOutMin=[]  UintegralTsProdOutMax=[]  UngainTsProdOutMin=[]  UngainTsProdOutMax=[]  IntegratorContinuousStateAttributes=''  IntegratorStateMustResolveToSignalObject=off  IntegratorRTWStateStorageClass=Auto  FilterContinuousStateAttributes=''  FilterStateMustResolveToSignalObject=off  FilterRTWStateStorageClass=Auto  ParallelPVariant=InternalParameters  IdealPVariant=Disabled  IVariant=InternalParameters  DVariant=InternalParameters  IntegratorVariant=Discrete  SatVariant=Disabled  AWVariant=Passthrough  PCopyVariant=Disabled  TRVariant=Disabled  FdbkBlocksVariant=Forward  IdealPFdbkVariant=Disabled  SatFdbkVariant=Disabled  DerivativeFilterVariant=ForwardEulerFilter  NVariant=InternalParameters  NCopyVariant=Disabled  FilterICVariant=InternalICsFilter  IntegratorICVariant=InternalICs  ExternalResetVariant=Disabled  TRSumVariant=Passthrough  SumFdbkVariant=Disabled  SumVariant=Sum_PID  TsampFilterVariant=InternalTs  TsampNgainVariant=Passthrough  TsampIntegralVariant=Passthrough  ExternalSaturationOutDataTypeStr=Inherit: Same as second input
  emi_389 : simulink/Discontinuities/Wrap To Zero  Threshold=255
      settings: SourceProductBaseCode=SL
  emi_390 : VariablePulseGenerator  SampleTime=0.1
  emi_391 : Product  Inputs=*
  emi_393 : Gain
  emi_394 : RateLimiter  SampleTimeMode=inherited
  emi_395 : Rounding
  emi_396 : simulink/Discontinuities/PWM  DisableCoverage=on  Period=1  DisallowZeroDutyCycle=off  RunAtFixedTimeIntervals=off  SampleTime=0.1
  emi_397 : Sin  TimeSource=Use external signal  SampleTime=0
  emi_398 : DiscreteFir
  emi_399 : Sum  Inputs=+
  emi_400 : DeadZone  SaturateOnIntegerOverflow=on
  emi_401 : simulink/Discontinuities/PWM  DisableCoverage=on  Period=1  DisallowZeroDutyCycle=off  RunAtFixedTimeIntervals=off  SampleTime=0.1
  emi_402 : DiscreteZeroPole  Poles=[0 0.5]  Gain=1  SampleTime=-1
  emi_403 : Sin  TimeSource=Use external signal  SampleTime=0
  emi_404 : simulink/Sources/Repeating Sequence  rep_seq_t=[0 2]  rep_seq_y=[0 2]
  Out1 : Outport
  emi_369 : Outport  Port=2
  wires:
  In1/1 -> Out1/1
  emi_370/1 -> emi_371/1
  emi_371/1 -> emi_372/1
  emi_372/1 -> emi_373/1
  emi_373/1 -> emi_374/1
  emi_374/1 -> emi_375/1
  emi_375/1 -> emi_376/1
  emi_376/1 -> emi_377/1
  emi_377/1 -> emi_378/1
  emi_378/1 -> emi_379/1
  emi_379/1 -> emi_380/1
  emi_380/1 -> emi_381/1
  emi_381/1 -> emi_382/1
  emi_382/1 -> emi_383/1
  emi_383/1 -> emi_384/1
  emi_384/1 -> emi_385/1
  emi_385/1 -> emi_386/1
  emi_386/1 -> emi_387/1
  emi_387/1 -> emi_388/1
  emi_388/1 -> emi_389/1
  emi_389/1 -> emi_390/1
  emi_390/1 -> emi_391/1
  emi_391/1 -> emi_392/1
  emi_392/1 -> emi_393/1
  emi_393/1 -> emi_394/1
  emi_394/1 -> emi_395/1
  emi_395/1 -> emi_396/1
  emi_396/1 -> emi_397/1
  emi_397/1 -> emi_398/1
  emi_398/1 -> emi_399/1
  emi_399/1 -> emi_400/1
  emi_400/1 -> emi_401/1
  emi_401/1 -> emi_402/1
  emi_402/1 -> emi_403/1
  emi_404/1 -> emi_370/1
  emi_403/1 -> emi_369/1

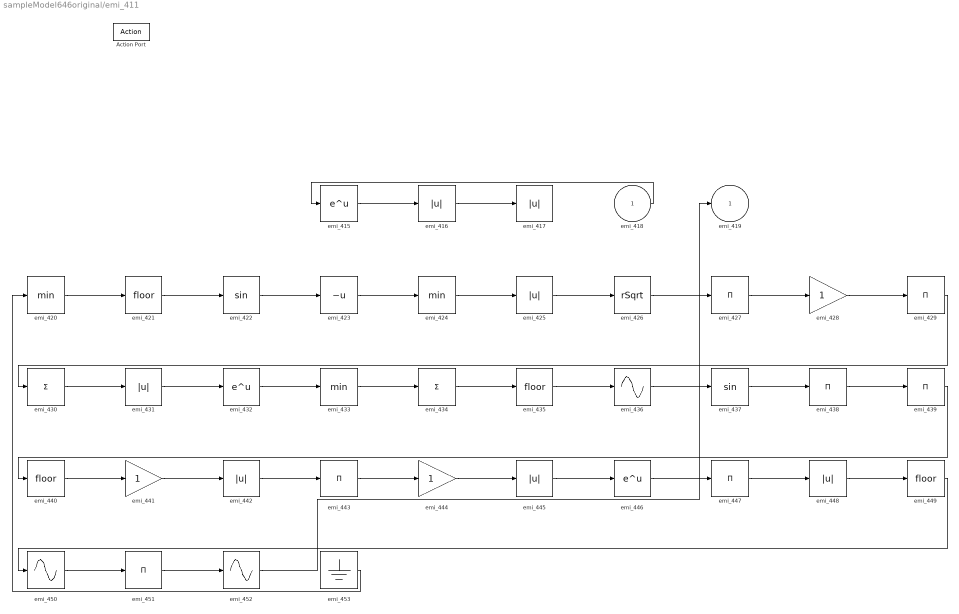
== system sampleModel646original/emi_411 ==
  emi_418 : Inport
  Action Port : ActionPort  ActionPortLabel=if(0 > u1)
  emi_415 : Math  SaturateOnIntegerOverflow=on
  emi_{416..417,425,431,442,445,448} (7 alike) : Abs
  emi_420 : MinMax
  emi_{421,435,440,449} (4 alike) : Rounding
  emi_422 : Trigonometry
  emi_423 : UnaryMinus
  emi_424 : MinMax
  emi_426 : Sqrt  Operator=rSqrt  SaturateOnIntegerOverflow=on
  emi_{427,429,438..439,443,447,451} (7 alike) : Product  Inputs=*
  emi_428 : Gain
  emi_430 : Sum  Inputs=+
  emi_432 : Math  SaturateOnIntegerOverflow=on
  emi_433 : MinMax
  emi_434 : Sum  Inputs=+
  emi_436 : Sin  TimeSource=Use external signal  SampleTime=0
  emi_437 : Trigonometry
  emi_441 : Gain
  emi_444 : Gain
  emi_446 : Math  SaturateOnIntegerOverflow=on
  emi_450 : Sin  TimeSource=Use external signal  SampleTime=0
  emi_452 : Sin  TimeSource=Use external signal  SampleTime=0
  emi_453 : Ground
  emi_419 : Outport
  wires:
  emi_418/1 -> emi_415/1
  emi_415/1 -> emi_416/1
  emi_416/1 -> emi_417/1
  emi_420/1 -> emi_421/1
  emi_421/1 -> emi_422/1
  emi_422/1 -> emi_423/1
  emi_423/1 -> emi_424/1
  emi_424/1 -> emi_425/1
  emi_425/1 -> emi_426/1
  emi_426/1 -> emi_427/1
  emi_427/1 -> emi_428/1
  emi_428/1 -> emi_429/1
  emi_429/1 -> emi_430/1
  emi_430/1 -> emi_431/1
  emi_431/1 -> emi_432/1
  emi_432/1 -> emi_433/1
  emi_433/1 -> emi_434/1
  emi_434/1 -> emi_435/1
  emi_435/1 -> emi_436/1
  emi_436/1 -> emi_437/1
  emi_437/1 -> emi_438/1
  emi_438/1 -> emi_439/1
  emi_439/1 -> emi_440/1
  emi_440/1 -> emi_441/1
  emi_441/1 -> emi_442/1
  emi_442/1 -> emi_443/1
  emi_443/1 -> emi_444/1
  emi_444/1 -> emi_445/1
  emi_445/1 -> emi_446/1
  emi_446/1 -> emi_447/1
  emi_447/1 -> emi_448/1
  emi_448/1 -> emi_449/1
  emi_449/1 -> emi_450/1
  emi_450/1 -> emi_451/1
  emi_451/1 -> emi_452/1
  emi_453/1 -> emi_420/1
  emi_452/1 -> emi_419/1

== system sampleModel646original/emi_456 ==
  In1 : Inport
  emi_457 : Inport  Port=2
  emi_459 : Sqrt  Operator=rSqrt  SaturateOnIntegerOverflow=on
  emi_460 : VariablePulseGenerator  SampleTime=0.1
  emi_461 : Subsystem  Tag=STV Subsys  LoadFcn=sigbuilder_block('load');  StartFcn=sigbuilder_block('start');  StopFcn=sigbuilder_block('stop');  ClipboardFcn=sigbuilder_block('clipboard');  mask(Sigbuilder block){tuvar=[0:10]}
      mask help: Simulink:masks:SigbuilderBlock_MD
      mask init:
      | if ~strcmp(get_param(bdroot(gcbh),'SimulationStatus'),'stopped') tuvar = sigbuilder_block('maskInit'); end
      settings: CopyFcn=sigbuilder_block('copy');  DeleteFcn=sigbuilder_block('delete');  ModelCloseFcn=sigbuilder_block('modelClose');  PreSaveFcn=sigbuilder_block('preSave');  PauseFcn=sigbuilder_block('pause');  ContinueFcn=sigbuilder_block('continue');  NameChangeFcn=sigbuilder_block('namechange');  OpenFcn=sigbuilder_block('open',[437.6 199.2 550.4 400 ]);  CloseFcn=sigbuilder_block('close');
      mask Display: plot(0, 0, 100, 100,[2, 2, 32, 32, 2], [68, 8, 8, 68, 68],[32, 2], [38, 38], [32, 19, 2],[53, 60, 44], [32, 17, 17, 2],[16, 16, 31, 31]);txt = getActiveGroup(gcbh);text(2, 100, txt,'verticalAlignment', 'top');
  Out1 : Outport
  emi_458 : Outport  Port=2
  wires:
  In1/1 -> Out1/1
  emi_459/1 -> emi_460/1
  emi_461/1(Signal 1) -> emi_459/1
  emi_460/1 -> emi_458/1

== system sampleModel646original/emi_468 ==
  emi_475 : Inport
  Action Port : ActionPort  ActionPortLabel=if(-1.617560e+02 > u1)
  emi_472 : Gain
  emi_473 : Abs
  emi_474 : Math  SaturateOnIntegerOverflow=on
  emi_477 : Trigonometry
  emi_478 : Sin  TimeSource=Use external signal  SampleTime=0
  emi_{479,481,483..485,489,500} (7 alike) : UnaryMinus
  emi_480 : MinMax
  emi_482 : Sum  Inputs=+
  emi_486 : Product  Inputs=*
  emi_487 : Abs
  emi_488 : MinMax
  emi_490 : Trigonometry
  emi_491 : Sum  Inputs=+
  emi_492 : MinMax
  emi_493 : Math  SaturateOnIntegerOverflow=on
  emi_494 : Gain
  emi_495 : Sin  TimeSource=Use external signal  SampleTime=0
  emi_496 : Sqrt  Operator=rSqrt  SaturateOnIntegerOverflow=on
  emi_497 : Math  SaturateOnIntegerOverflow=on
  emi_498 : Product  Inputs=*
  emi_499 : Sin  TimeSource=Use external signal  SampleTime=0
  emi_501 : Product  Inputs=*
  emi_502 : Gain
  emi_503 : Ground
  emi_476 : Outport
  wires:
  emi_475/1 -> emi_472/1
  emi_472/1 -> emi_473/1
  emi_473/1 -> emi_474/1
  emi_477/1 -> emi_478/1
  emi_478/1 -> emi_479/1
  emi_479/1 -> emi_480/1
  emi_480/1 -> emi_481/1
  emi_481/1 -> emi_482/1
  emi_482/1 -> emi_483/1
  emi_483/1 -> emi_484/1
  emi_484/1 -> emi_485/1
  emi_485/1 -> emi_486/1
  emi_486/1 -> emi_487/1
  emi_487/1 -> emi_488/1
  emi_488/1 -> emi_489/1
  emi_489/1 -> emi_490/1
  emi_490/1 -> emi_491/1
  emi_491/1 -> emi_492/1
  emi_492/1 -> emi_493/1
  emi_493/1 -> emi_494/1
  emi_494/1 -> emi_495/1
  emi_495/1 -> emi_496/1
  emi_496/1 -> emi_497/1
  emi_497/1 -> emi_498/1
  emi_498/1 -> emi_499/1
  emi_499/1 -> emi_500/1
  emi_500/1 -> emi_501/1
  emi_501/1 -> emi_502/1
  emi_503/1 -> emi_477/1
  emi_502/1 -> emi_476/1
